simulink model "ClosedLoop_old"  (R2023a)
settings: Solver=FixedStepAuto  StartTime=0.0  StopTime=34.4428  FixedStep=0.001  RelTol=1e-3  EnableMultiTasking=on
values from neighbouring files (symbols this model uses):
  x0 = [-pi/2;0;0;0]    [MAIN.m]    (also in MAIN_HW.m; fitParams.m = [-pi/2; 0; 0; 0])
undefined symbols (not defined in the file or in its folder): DiscIntNeverNeededParam
libraries: simulink x2
settings Model: ExtModeTrigType=signal  ExtModeTrigDuration=60000  ExtModeTrigDirection=either  ExtModeTrigLevel=0.500000  Creator=colegiusto  LastModifiedBy=colegiusto
settings SolverCC: PositivePriorityOrder=on
settings OptimizationCC: BlockReduction=off  DefaultParameterBehavior=Inlined  BufferReuse=off
settings RTWCC: Description=QUARC Win64 Target Using Toolchain  SystemTargetFile=quarc_win64.tlc  Toolchain=QUARC win64 | nmake (64-bit Windows)  BuildConfiguration=Faster Runs
settings STFCustomTargetCC: TargetLangStandard=C89/C90 (ANSI)  SystemTargetFile=quarc_win64.tlc
settings GRTTargetCC: TargetLangStandard=C89/C90 (ANSI)  ParMdlRefBuildCompliant=off  CompOptLevelCompliant=off  CombineOutputUpdateFcns=off  MatFileLogging=off  CPPClassGenCompliant=off  GRTInterface=on  ExtMode=on  ExtModeMexFile=quarc_comm

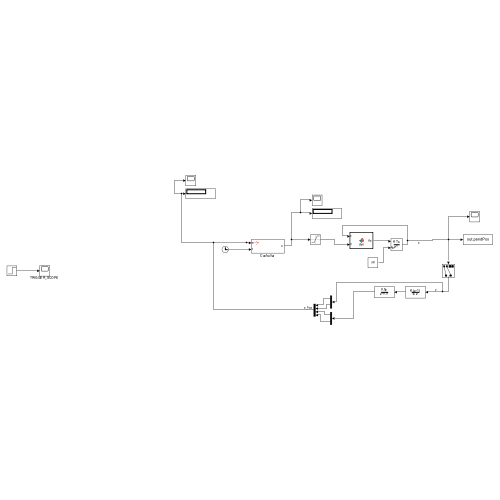
[thumbnail: Simulink's stored preview of the top-level diagram]
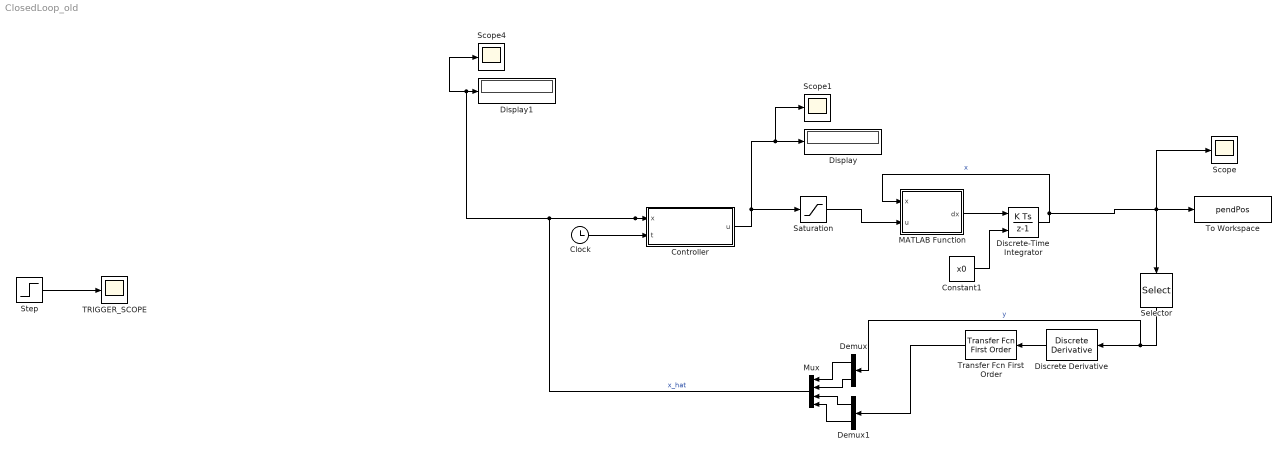
== system ClosedLoop_old ==
  Clock : Clock
  Constant1 : Constant  Value=x0  VectorParams1D=off
  Controller : Subsystem
  Demux : Demux  Outputs=2
  Demux1 : Demux  Outputs=2
  Discrete Derivative : simulink/Discrete/Discrete Derivative  gainval=1.0  ICPrevScaledInput=0.0  OutMin=[]  OutMax=[]  OutDataType=fixdt(1, 16)  OutScaling=2^-10  DoSatur=off
  Discrete-Time Integrator : DiscreteIntegrator  InitialConditionSource=external  SampleTime=-1  ICPrevOutput=DiscIntNeverNeededParam  ICPrevScaledInput=DiscIntNeverNeededParam
  Display : Display
  Display1 : Display
  MATLAB Function : MATLAB Function  TreatAsAtomicUnit=on
  Mux : Mux
  Saturation : Saturate  UpperLimit=5  LowerLimit=-5
  Scope : Scope
  Scope1 : Scope
  Scope4 : Scope
  Selector : Selector  InputPortWidth=4  IndexOptions=Index vector (dialog)  Indices=[1,2]  OutputSizes=1
  Step : Step  Time=0.001  SampleTime=0
  TRIGGER_SCOPE : Scope
  To Workspace : ToWorkspace  VariableName=pendPos  SaveFormat=Structure With Time  SampleTime=-1
  Transfer Fcn First Order : simulink/Discrete/Transfer Fcn First Order  PoleZ=0.5  ICPrevOutput=0.0  DoSatur=off
  wires:
  Step/1 -> TRIGGER_SCOPE/1
  Saturation/1 -> MATLAB Function/2(u)
  Constant1/1 -> Discrete-Time Integrator/2
  MATLAB Function/1(dx) -> Discrete-Time Integrator/1
  Discrete-Time Integrator/1 -> MATLAB Function/1(x), Selector/1, Scope/1, To Workspace/1  "x"
  Selector/1 -> Demux/1, Discrete Derivative/1  "y"
  Discrete Derivative/1 -> Transfer Fcn First Order/1
  Demux/1 -> Mux/1
  Demux/2 -> Mux/2
  Demux1/1 -> Mux/3
  Demux1/2 -> Mux/4
  Mux/1 -> Controller/1(x), Scope4/1, Display1/1  "x_hat"
  Clock/1 -> Controller/2(t)
  Controller/1(u) -> Scope1/1, Display/1, Saturation/1
  Transfer Fcn First Order/1 -> Demux1/1

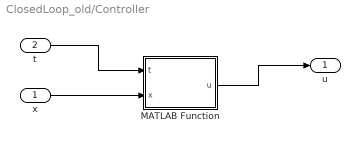
== system ClosedLoop_old/Controller ==
  x : Inport
  t : Inport  Port=2
  MATLAB Function : MATLAB Function  TreatAsAtomicUnit=on
  u : Outport
  wires:
  x/1 -> MATLAB Function/2(x)
  MATLAB Function/1(u) -> u/1
  t/1 -> MATLAB Function/1(t)

== matlab function ClosedLoop_old/Controller/MATLAB Function ==
  data: t input; x input; u output; c parameter
function u = linearController(t, x, c)
u = linearControl(t, x, c);

== matlab function ClosedLoop_old/MATLAB Function ==
  data: x input; u input; dx output; p parameter
function dx = dyn(x,u,p)
    dx = dynamics(x,u,p);
end
